simulink model "slip_torque_host"  (R2021b)
settings: Solver=FixedStepAuto  StartTime=0.0  StopTime=inf  FixedStep=1e-3  RelTol=1e-3
libraries: slrealtimeutilitieslib x1, slrealtimeiplib x1
settings Model: Creator=tcraddoc  LastModifiedBy=wasynczu
settings SolverCC: AlgebraicLoopSolver=TrustRegion
settings DataIOCC: ReturnWorkspaceOutputs=off
settings DebuggingCC: SFMachineParentedDataDiag=warning  ArithmeticOperatorsInVariantConditions=warning
settings SFSimCC: SimUseLocalCustomCode=off  CustomCodeUndefinedFunction=UseInterfaceOnly
settings RTWCC: RTWUseLocalCustomCode=off
settings CodeAppCC: StateflowObjectComments=on

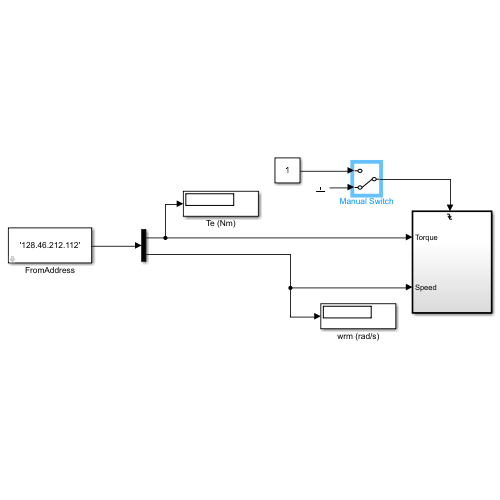
[thumbnail: Simulink's stored preview of the top-level diagram]
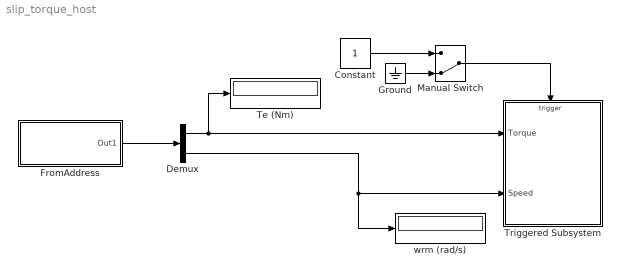
== system slip_torque_host ==
  Constant : Constant
  Demux : Demux  Outputs=2
  FromAddress : Subsystem  mask{fromIPAddress='128.46.212.112'}
      mask prompts: fromIPAddress "From IP Address"
      mask Display: disp((get_param(gcb,'fromIPAddress')))
  Ground : Ground
  Manual Switch : ManualSwitch  CurrentSetting=0
  Te (Nm) : Display
  Triggered Subsystem : Subsystem  TreatAsAtomicUnit=on
  wrm (rad/s) : Display
  wires:
  Demux/2 -> Triggered Subsystem/2(Speed), wrm (rad/s)/1
  Demux/1 -> Triggered Subsystem/1(Torque), Te (Nm)/1
  Constant/1 -> Manual Switch/1
  Ground/1 -> Manual Switch/2
  Manual Switch/1 -> Triggered Subsystem/Trigger
  FromAddress/1(Out1) -> Demux/1

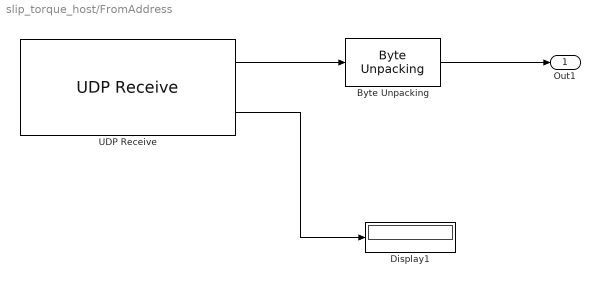
== system slip_torque_host/FromAddress ==
  Byte Unpacking : slrealtimeutilitieslib/Byte Unpacking  MaskUnpackedDataTypes={['double']}  MaskUnpackedDataSizes={[2]}  MaskAlignment=1
      settings: SourceProductBaseCode=XP
  Display1 : Display
  UDP Receive : slrealtimeiplib/UDP Receive  useHostTargetConn=on  ipAddress=128.46.212.188  localPort=34  rcvWidth=16  rcvFmAny=off  fmAddress=fromIPAddress  sampleTime=1e-3
      settings: SourceProductBaseCode=XP
  Out1 : Outport
  wires:
  Byte Unpacking/1 -> Out1/1
  UDP Receive/2 -> Display1/1
  UDP Receive/1 -> Byte Unpacking/1

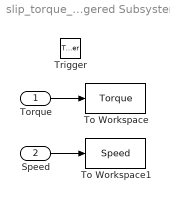
== system slip_torque_host/Triggered Subsystem ==
  Torque : Inport
  Speed : Inport  Port=2
  Trigger : TriggerPort  TriggerType=falling  VariantControl=Variant
  To Workspace : ToWorkspace  VariableName=Torque  SampleTime=-1
  To Workspace1 : ToWorkspace  VariableName=Speed  SampleTime=-1
  wires:
  Torque/1 -> To Workspace/1
  Speed/1 -> To Workspace1/1
